simulink model "orthographic_projection_sfchart_tb"  (R2018b)
settings: Solver=FixedStepDiscrete  StartTime=0.0  StopTime=inf  FixedStep=1  RelTol=1e-3
undefined symbols (not defined in the file): lambda0Val, lambdaVec, nIters, numSamples, phi0Val, phiVec, RE
libraries: hdlsllib x10, cordic_rotation_mode x2, simulink x1
settings Model: DataTypeOverride=Off  Creator=jimjoy  LastModifiedBy=tbryan
settings DataIOCC: SaveFormat=StructureWithTime  SaveOutput=off  DSMLogging=off  SaveTime=off  ReturnWorkspaceOutputs=on
settings OptimizationCC: BlockReduction=off  ConditionallyExecuteInputs=off  DefaultParameterBehavior=Inlined
settings DebuggingCC: AlgebraicLoopMsg=error  SingleTaskRateTransMsg=error  UnderSpecifiedDataTypeMsg=error  UnderSpecifiedDimensionMsg=error
settings HardwareCC: ProdBitPerPointer=32  ProdBitPerSizeT=32  ProdBitPerPtrDiffT=32  ProdLargestAtomicFloat=None  ProdIntDivRoundTo=Undefined  ProdEndianess=Unspecified  ProdWordSize=32  ProdHWDeviceType=ASIC/FPGA->ASIC/FPGA  TargetBitPerLong=64  TargetBitPerPointer=64  TargetBitPerSizeT=64  TargetBitPerPtrDiffT=64  TargetLongLongMode=on  TargetIntDivRoundTo=Zero  TargetEndianess=LittleEndian  TargetWordSize=64  TargetHWDeviceType=Custom Processor->MATLAB Host Computer  ProdEqTarget=off

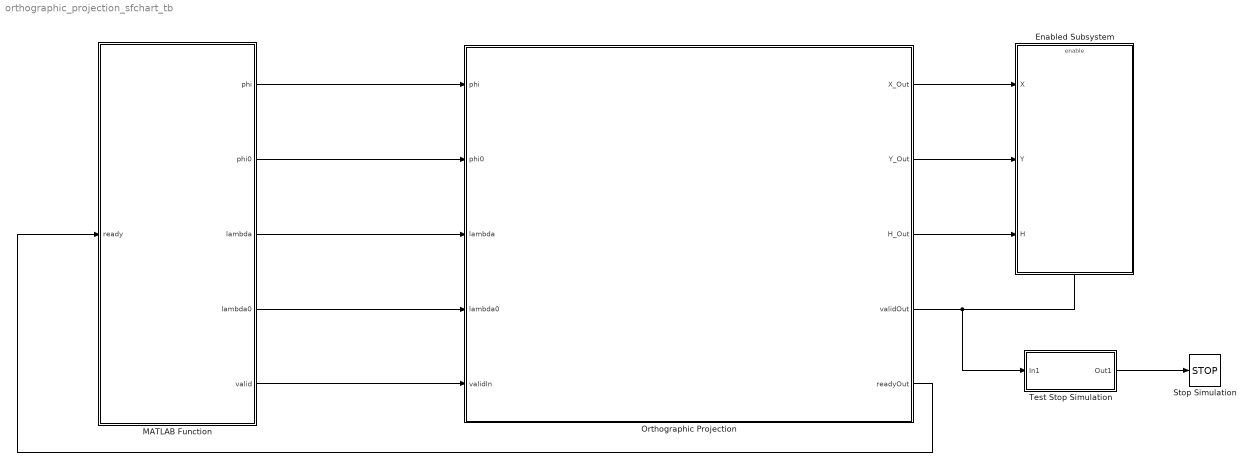
== system orthographic_projection_sfchart_tb ==
  Enabled Subsystem : Subsystem  TreatAsAtomicUnit=on
  MATLAB Function : MATLAB Function  TreatAsAtomicUnit=on  mask{phiVec=phiVec, lambdaVec=lambdaVec, phi0Val=phi0Val, lambda0Val=lambda0Val}
      mask prompts: phiVec "phi"; lambdaVec "lambda"; phi0Val "phi0"; lambda0Val "lambda0"
  Orthographic Projection : Subsystem
  Stop Simulation : Stop
  Test Stop Simulation : Subsystem
  wires:
  Orthographic Projection/1(X_Out) -> Enabled Subsystem/1(X)
  Orthographic Projection/2(Y_Out) -> Enabled Subsystem/2(Y)
  Orthographic Projection/3(H_Out) -> Enabled Subsystem/3(H)
  Orthographic Projection/4(validOut) -> Test Stop Simulation/1(In1), Enabled Subsystem/Enable
  Orthographic Projection/5(readyOut) -> MATLAB Function/1(ready)
  MATLAB Function/5(valid) -> Orthographic Projection/5(validIn)
  MATLAB Function/4(lambda0) -> Orthographic Projection/4(lambda0)
  MATLAB Function/3(lambda) -> Orthographic Projection/3(lambda)
  MATLAB Function/2(phi0) -> Orthographic Projection/2(phi0)
  Test Stop Simulation/1(Out1) -> Stop Simulation/1
  MATLAB Function/1(phi) -> Orthographic Projection/1(phi)

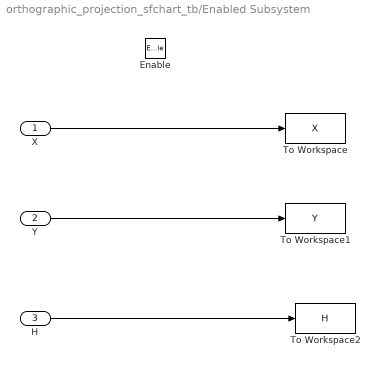
== system orthographic_projection_sfchart_tb/Enabled Subsystem ==
  X : Inport
  Y : Inport  Port=2
  H : Inport  Port=3
  Enable : EnablePort
  To Workspace : ToWorkspace  VariableName=X  SampleTime=-1
      settings: Save2DSignal=2-D array (concatenate along first dimension)
  To Workspace1 : ToWorkspace  VariableName=Y  SampleTime=-1
      settings: Save2DSignal=2-D array (concatenate along first dimension)
  To Workspace2 : ToWorkspace  VariableName=H  SampleTime=-1
      settings: Save2DSignal=2-D array (concatenate along first dimension)
  wires:
  X/1 -> To Workspace/1
  Y/1 -> To Workspace1/1
  H/1 -> To Workspace2/1

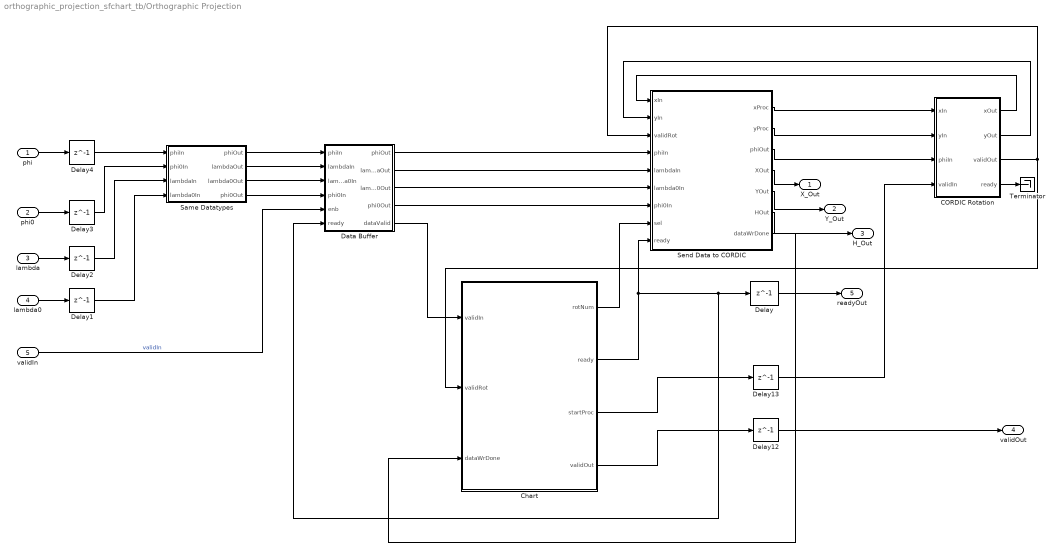
== system orthographic_projection_sfchart_tb/Orthographic Projection ==
  phi : Inport
  phi0 : Inport  Port=2
  lambda : Inport  Port=3
  lambda0 : Inport  Port=4
  validIn : Inport  Port=5
  CORDIC Rotation : Subsystem
  Chart : Stateflow chart  TreatAsAtomicUnit=on
  Data Buffer : Subsystem
  Delay{,1..4,12..13} (7 alike) : Delay  DelayLength=1
  Same Datatypes : Subsystem
  Send Data to CORDIC : Subsystem
  Terminator : Terminator
  X_Out : Outport
  Y_Out : Outport  Port=2
  H_Out : Outport  Port=3
  validOut : Outport  Port=4
  readyOut : Outport  Port=5
  wires:
  CORDIC Rotation/3(validOut) -> Chart/2(validRot), Send Data to CORDIC/3(validRot)
  Chart/4(validOut) -> Delay12/1
  lambda0/1 -> Delay1/1
  phi0/1 -> Delay3/1
  lambda/1 -> Delay2/1
  phi/1 -> Delay4/1
  Delay13/1 -> CORDIC Rotation/4(validIn)
  Send Data to CORDIC/3(phiOut) -> CORDIC Rotation/3(phiIn)
  Send Data to CORDIC/2(yProc) -> CORDIC Rotation/2(yIn)
  Send Data to CORDIC/1(xProc) -> CORDIC Rotation/1(xIn)
  CORDIC Rotation/4(ready) -> Terminator/1
  Delay12/1 -> validOut/1
  Same Datatypes/1(phiOut) -> Data Buffer/1(phiIn)
  Same Datatypes/2(lambdaOut) -> Data Buffer/2(lambdaIn)
  Same Datatypes/3(lambda0Out) -> Data Buffer/3(lambda0In)
  Same Datatypes/4(phi0Out) -> Data Buffer/4(phi0In)
  Delay1/1 -> Same Datatypes/4(lambda0In)
  Delay2/1 -> Same Datatypes/3(lambdaIn)
  Delay3/1 -> Same Datatypes/2(phi0In)
  Delay4/1 -> Same Datatypes/1(phiIn)
  Chart/3(startProc) -> Delay13/1
  CORDIC Rotation/1(xOut) -> Send Data to CORDIC/1(xIn)
  Data Buffer/1(phiOut) -> Send Data to CORDIC/4(phiIn)
  Data Buffer/2(lambdaOut) -> Send Data to CORDIC/5(lambdaIn)
  Data Buffer/3(lambda0Out) -> Send Data to CORDIC/6(lambda0In)
  Data Buffer/4(phi0Out) -> Send Data to CORDIC/7(phi0In)
  CORDIC Rotation/2(yOut) -> Send Data to CORDIC/2(yIn)
  Chart/1(rotNum) -> Send Data to CORDIC/8("sel ")
  Send Data to CORDIC/4(XOut) -> X_Out/1
  Send Data to CORDIC/5(YOut) -> Y_Out/1
  Send Data to CORDIC/6(HOut) -> H_Out/1
  validIn/1 -> Data Buffer/5(enb)  "validIn"
  Data Buffer/5(dataValid) -> Chart/1(validIn)
  Chart/2(ready) -> Data Buffer/6(ready), Delay/1, Send Data to CORDIC/9(ready)
  Delay/1 -> readyOut/1
  Send Data to CORDIC/7(dataWrDone) -> Chart/3(dataWrDone)

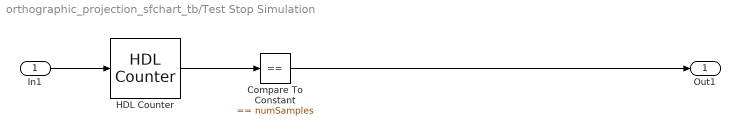
== system orthographic_projection_sfchart_tb/Test Stop Simulation ==
  In1 : Inport
  Compare To Constant : simulink/Logic and Bit Operations/Compare To Constant  relop===  const=numSamples  OutDataTypeStr=boolean
  HDL Counter : hdlsllib/Sources/HDL Counter  CountType=Free running  CountInit=0  CountStep=1  CountMax=25  CountFromType=Initial value  CountFrom=0  CountResetPort=off  CountLoadPort=off  CountEnbPort=on  CountDirPort=off  CountDataType=Unsigned  CountWordLen=nextpow2(numSamples)  CountFracLen=0  CountSampTime=1
      settings: SourceProductName=Simulink
  Out1 : Outport
  wires:
  In1/1 -> HDL Counter/1
  HDL Counter/1 -> Compare To Constant/1
  Compare To Constant/1 -> Out1/1

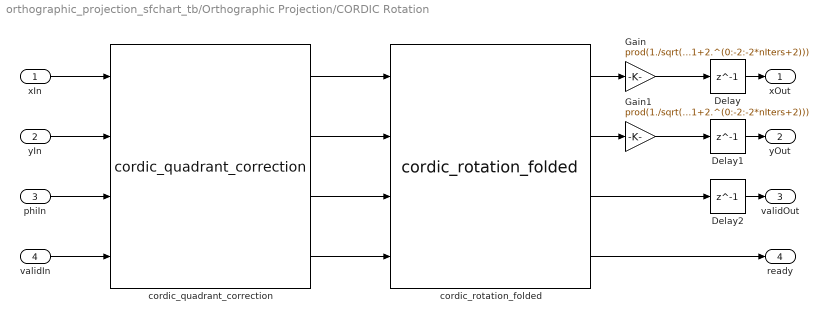
== system orthographic_projection_sfchart_tb/Orthographic Projection/CORDIC Rotation ==
  xIn : Inport
  yIn : Inport  Port=2
  phiIn : Inport  Port=3
  validIn : Inport  Port=4
  Delay : Delay  DelayLength=1
  Delay1 : Delay  DelayLength=1
  Delay2 : Delay  DelayLength=1
  Gain : Gain  Gain=prod(1./sqrt(1+2.^(0:-2:-2*nIters+2)))  OutDataTypeStr=Inherit: Same as input
  Gain1 : Gain  Gain=prod(1./sqrt(1+2.^(0:-2:-2*nIters+2)))  OutDataTypeStr=Inherit: Same as input
  cordic_quadrant_correction : cordic_rotation_mode/cordic_quadrant_correction  SystemSampleTime=-1
  cordic_rotation_folded : cordic_rotation_mode/cordic_rotation_folded  SystemSampleTime=-1
  xOut : Outport
  yOut : Outport  Port=2
  validOut : Outport  Port=3
  ready : Outport  Port=4
  wires:
  Gain1/1 -> Delay1/1
  cordic_quadrant_correction/1 -> cordic_rotation_folded/1
  cordic_rotation_folded/3 -> Delay2/1
  cordic_rotation_folded/2 -> Gain1/1
  cordic_rotation_folded/1 -> Gain/1
  cordic_quadrant_correction/2 -> cordic_rotation_folded/2
  cordic_quadrant_correction/3 -> cordic_rotation_folded/3
  Gain/1 -> Delay/1
  cordic_quadrant_correction/4 -> cordic_rotation_folded/4
  xIn/1 -> cordic_quadrant_correction/1
  Delay/1 -> xOut/1
  Delay2/1 -> validOut/1
  validIn/1 -> cordic_quadrant_correction/4
  Delay1/1 -> yOut/1
  phiIn/1 -> cordic_quadrant_correction/3
  yIn/1 -> cordic_quadrant_correction/2
  cordic_rotation_folded/4 -> ready/1

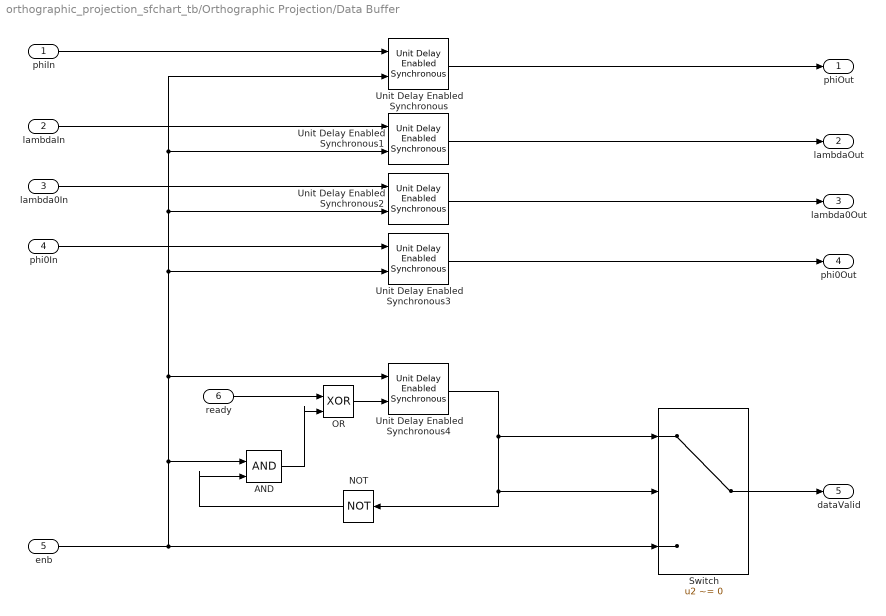
== system orthographic_projection_sfchart_tb/Orthographic Projection/Data Buffer ==
  phiIn : Inport
  lambdaIn : Inport  Port=2
  lambda0In : Inport  Port=3
  phi0In : Inport  Port=4
  enb : Inport  Port=5
  ready : Inport  Port=6
  AND : Logic  IconShape=distinctive  AllPortsSameDT=off  OutDataTypeStr=boolean
  NOT : Logic  Operator=NOT  IconShape=distinctive  AllPortsSameDT=off  OutDataTypeStr=boolean
  OR : Logic  Operator=XOR  IconShape=distinctive  AllPortsSameDT=off  OutDataTypeStr=boolean
  Switch : Switch  Criteria=u2 ~= 0
  Unit Delay Enabled Synchronous{,1..4} (5 alike) : hdlsllib/Discrete/Unit Delay Enabled Synchronous  InitialCondition=0.0  SampleTime=-1
      settings: SourceProductName=Simulink  SourceProductBaseCode=SL
  phiOut : Outport
  lambdaOut : Outport  Port=2
  lambda0Out : Outport  Port=3
  phi0Out : Outport  Port=4
  dataValid : Outport  Port=5
  wires:
  phiIn/1 -> Unit Delay Enabled Synchronous/1
  lambdaIn/1 -> Unit Delay Enabled Synchronous1/1
  lambda0In/1 -> Unit Delay Enabled Synchronous2/1
  phi0In/1 -> Unit Delay Enabled Synchronous3/1
  enb/1 -> AND/1, Unit Delay Enabled Synchronous4/1, Unit Delay Enabled Synchronous3/2, Unit Delay Enabled Synchronous2/2, Unit Delay Enabled Synchronous1/2, Unit Delay Enabled Synchronous/2, Switch/3
  Unit Delay Enabled Synchronous/1 -> phiOut/1
  Unit Delay Enabled Synchronous1/1 -> lambdaOut/1
  Unit Delay Enabled Synchronous2/1 -> lambda0Out/1
  Unit Delay Enabled Synchronous3/1 -> phi0Out/1
  Unit Delay Enabled Synchronous4/1 -> NOT/1, Switch/2, Switch/1
  ready/1 -> OR/1
  OR/1 -> Unit Delay Enabled Synchronous4/2
  AND/1 -> OR/2
  NOT/1 -> AND/2
  Switch/1 -> dataValid/1

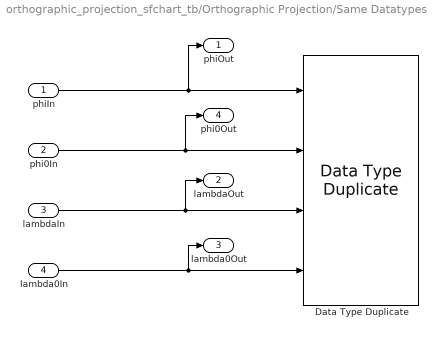
== system orthographic_projection_sfchart_tb/Orthographic Projection/Same Datatypes ==
  phiIn : Inport
  phi0In : Inport  Port=2
  lambdaIn : Inport  Port=3
  lambda0In : Inport  Port=4
  Data Type Duplicate : DataTypeDuplicate  NumInputPorts=4
  phiOut : Outport
  lambdaOut : Outport  Port=2
  lambda0Out : Outport  Port=3
  phi0Out : Outport  Port=4
  wires:
  lambdaIn/1 -> lambdaOut/1, Data Type Duplicate/3
  phiIn/1 -> Data Type Duplicate/1, phiOut/1
  lambda0In/1 -> lambda0Out/1, Data Type Duplicate/4
  phi0In/1 -> phi0Out/1, Data Type Duplicate/2

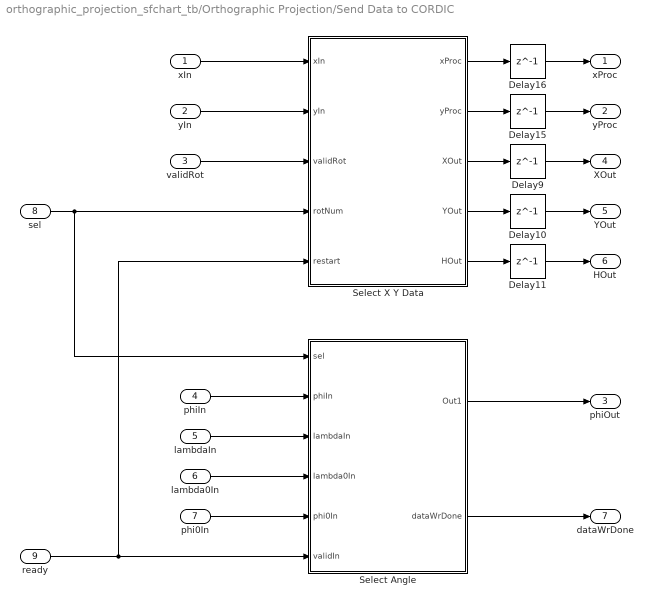
== system orthographic_projection_sfchart_tb/Orthographic Projection/Send Data to CORDIC ==
  xIn : Inport
  yIn : Inport  Port=2
  validRot : Inport  Port=3
  phiIn : Inport  Port=4
  lambdaIn : Inport  Port=5
  lambda0In : Inport  Port=6
  phi0In : Inport  Port=7
  "sel " : Inport  Port=8
  ready : Inport  Port=9
  Delay{9..11,15..16} (5 alike) : Delay  DelayLength=1
  Select Angle : Subsystem
  Select X Y Data : Subsystem  mask{RE=RE}
      mask prompts: RE "Radius of the Earth"
  xProc : Outport
  yProc : Outport  Port=2
  phiOut : Outport  Port=3
  XOut : Outport  Port=4
  YOut : Outport  Port=5
  HOut : Outport  Port=6
  dataWrDone : Outport  Port=7
  wires:
  "sel "/1 -> Select Angle/1(sel), Select X Y Data/4(rotNum)
  ready/1 -> Select X Y Data/5(restart), Select Angle/6("validIn ")
  phiIn/1 -> Select Angle/2(phiIn)
  lambdaIn/1 -> Select Angle/3(lambdaIn)
  lambda0In/1 -> Select Angle/4(lambda0In)
  phi0In/1 -> Select Angle/5(phi0In)
  Select X Y Data/1(xProc) -> Delay16/1
  xIn/1 -> Select X Y Data/1(xIn)
  Select X Y Data/2(yProc) -> Delay15/1
  yIn/1 -> Select X Y Data/2(yIn)
  validRot/1 -> Select X Y Data/3(validRot)
  Select X Y Data/3(XOut) -> Delay9/1
  Select X Y Data/5(HOut) -> Delay11/1
  Select X Y Data/4(YOut) -> Delay10/1
  Delay10/1 -> YOut/1
  Delay9/1 -> XOut/1
  Delay11/1 -> HOut/1
  Delay16/1 -> xProc/1
  Delay15/1 -> yProc/1
  Select Angle/1(Out1) -> phiOut/1
  Select Angle/2(dataWrDone) -> dataWrDone/1

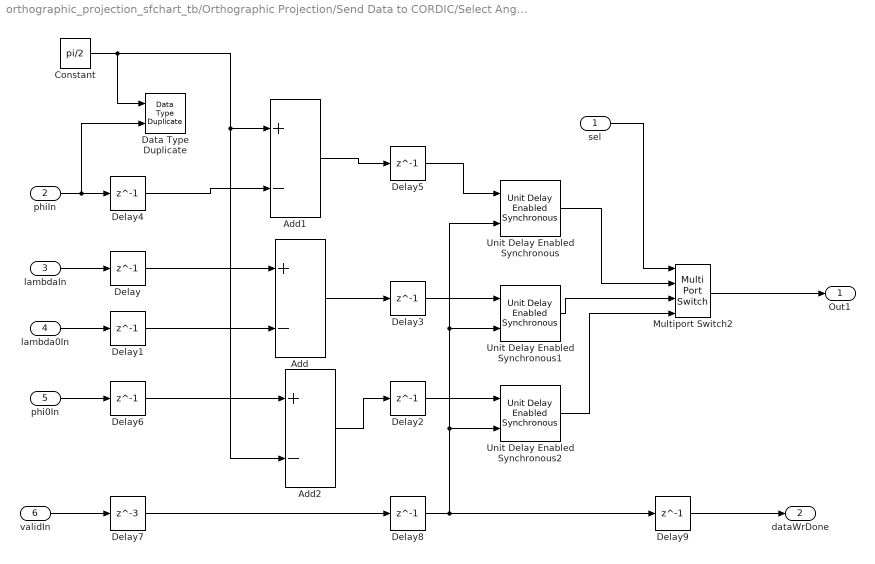
== system orthographic_projection_sfchart_tb/Orthographic Projection/Send Data to CORDIC/Select Angle ==
  sel : Inport
  phiIn : Inport  Port=2
  lambdaIn : Inport  Port=3
  lambda0In : Inport  Port=4
  phi0In : Inport  Port=5
  "validIn " : Inport  Port=6
  Add : Sum  Inputs=+-
  Add1 : Sum  Inputs=+-
  Add2 : Sum  Inputs=+-
  Constant : Constant  Value=pi/2  OutDataTypeStr=Inherit: Inherit via back propagation
  Data Type Duplicate : DataTypeDuplicate
  Delay{,1..6,8..9} (9 alike) : Delay  DelayLength=1
  Delay7 : Delay  DelayLength=3
  Multiport Switch2 : MultiPortSwitch  DataPortOrder=Zero-based contiguous  zeroidx=on
  Unit Delay Enabled Synchronous : hdlsllib/Discrete/Unit Delay Enabled Synchronous  InitialCondition=0.0  SampleTime=-1
      settings: SourceProductName=Simulink  SourceProductBaseCode=SL
  Unit Delay Enabled Synchronous1 : hdlsllib/Discrete/Unit Delay Enabled Synchronous  InitialCondition=0.0  SampleTime=-1
      settings: SourceProductName=Simulink  SourceProductBaseCode=SL
  Unit Delay Enabled Synchronous2 : hdlsllib/Discrete/Unit Delay Enabled Synchronous  InitialCondition=0.0  SampleTime=-1
      settings: SourceProductName=Simulink  SourceProductBaseCode=SL
  Out1 : Outport
  dataWrDone : Outport  Port=2
  wires:
  Unit Delay Enabled Synchronous/1 -> Multiport Switch2/2
  Unit Delay Enabled Synchronous1/1 -> Multiport Switch2/3
  Unit Delay Enabled Synchronous2/1 -> Multiport Switch2/4
  Multiport Switch2/1 -> Out1/1
  sel/1 -> Multiport Switch2/1
  "validIn "/1 -> Delay7/1
  phi0In/1 -> Delay6/1
  phiIn/1 -> Data Type Duplicate/2, Delay4/1
  lambdaIn/1 -> Delay/1
  lambda0In/1 -> Delay1/1
  Delay/1 -> Add/1
  Delay1/1 -> Add/2
  Add/1 -> Delay3/1
  Add2/1 -> Delay2/1
  Delay2/1 -> Unit Delay Enabled Synchronous2/1
  Delay3/1 -> Unit Delay Enabled Synchronous1/1
  Delay5/1 -> Unit Delay Enabled Synchronous/1
  Delay6/1 -> Add2/1
  Delay7/1 -> Delay8/1
  Delay8/1 -> Delay9/1, Unit Delay Enabled Synchronous/2, Unit Delay Enabled Synchronous1/2, Unit Delay Enabled Synchronous2/2
  Delay9/1 -> dataWrDone/1
  Delay4/1 -> Add1/2
  Add1/1 -> Delay5/1
  Constant/1 -> Data Type Duplicate/1, Add2/2, Add1/1

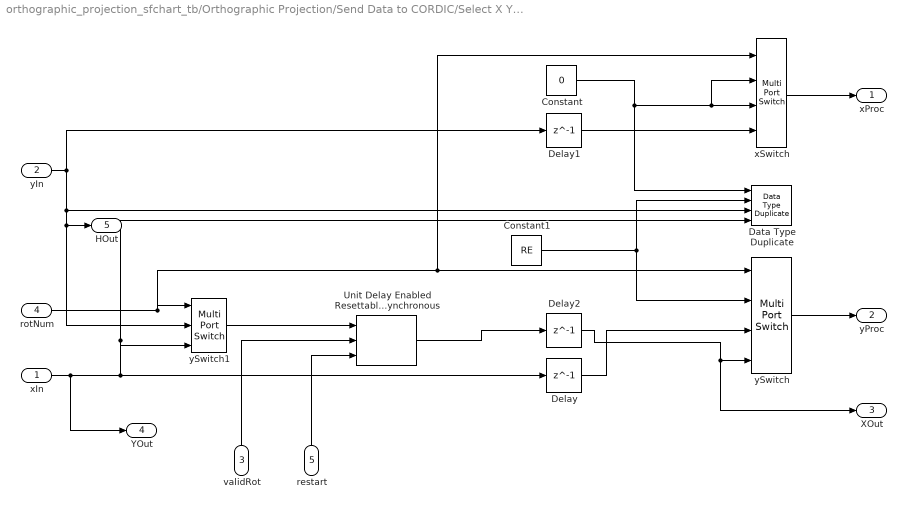
== system orthographic_projection_sfchart_tb/Orthographic Projection/Send Data to CORDIC/Select X Y Data ==
  xIn : Inport
  yIn : Inport  Port=2
  validRot : Inport  Port=3
  rotNum : Inport  Port=4
  restart : Inport  Port=5
  Constant : Constant  Value=0  OutDataTypeStr=Inherit: Inherit via back propagation
  Constant1 : Constant  Value=RE
  Data Type Duplicate : DataTypeDuplicate  NumInputPorts=4
  Delay : Delay  DelayLength=1
  Delay1 : Delay  DelayLength=1
  Delay2 : Delay  DelayLength=1
  Unit Delay Enabled Resettable Synchronous : hdlsllib/Discrete/Unit Delay Enabled Resettable Synchronous  InitialCondition=0.0  SampleTime=-1
      settings: SourceProductName=Simulink  SourceProductBaseCode=SL
  xSwitch : MultiPortSwitch  DataPortOrder=Zero-based contiguous  zeroidx=on
  ySwitch : MultiPortSwitch  DataPortOrder=Zero-based contiguous  zeroidx=on
  ySwitch1 : MultiPortSwitch  DataPortOrder=Zero-based contiguous  Inputs=2  DiagnosticForDefault=None  zeroidx=on
  xProc : Outport
  yProc : Outport  Port=2
  XOut : Outport  Port=3
  YOut : Outport  Port=4
  HOut : Outport  Port=5
  wires:
  ySwitch/1 -> yProc/1
  xSwitch/1 -> xProc/1
  Constant/1 -> Data Type Duplicate/1, xSwitch/3, xSwitch/2
  Constant1/1 -> Data Type Duplicate/2, ySwitch/2
  Unit Delay Enabled Resettable Synchronous/1 -> Delay2/1
  xIn/1 -> Data Type Duplicate/4, ySwitch1/3, Delay/1, YOut/1
  yIn/1 -> Data Type Duplicate/3, ySwitch1/2, HOut/1, Delay1/1
  ySwitch1/1 -> Unit Delay Enabled Resettable Synchronous/1
  rotNum/1 -> ySwitch1/1, ySwitch/1, xSwitch/1
  validRot/1 -> Unit Delay Enabled Resettable Synchronous/2
  restart/1 -> Unit Delay Enabled Resettable Synchronous/3
  Delay/1 -> ySwitch/3
  Delay1/1 -> xSwitch/4
  Delay2/1 -> XOut/1, ySwitch/4

== matlab function orthographic_projection_sfchart_tb/MATLAB Function ==
  data: ready input; phi output; phi0 output; lambda output; lambda0 output; valid output; phiVec parameter; lambdaVec parameter; numSamples parameter; phi0Val parameter; lambda0Val parameter
function [phi, phi0, lambda, lambda0, valid] = getData(ready, phiVec, lambdaVec, numSamples, phi0Val, lambda0Val)
%#codegen

persistent ii 

if isempty(ii)
    ii = 1;
end

phi0 = phi0Val;
lambda0 = lambda0Val;
phi = phiVec(ii);
lambda = lambdaVec(ii);

if ready
   valid = true;
   if ii < numSamples
      ii = ii + 1;
   else
       ii = 1;
   end
else
    valid = false;
end

end

== stateflow chart orthographic_projection_sfchart_tb/Orthographic Projection/Chart ==
  settings: stateMachineType=MEALY_MACHINE  executeAtInitialization=1
  state Controller
    state Init
    state Done
    state Idle
    state Processing
    state ProcessRotResults
    (default) -> Init : {ready = true;}
    Done -> Init : {rotNum = 0; ready = true;validOut = false;}
    Init -> Idle : [validIn]{ready = false;}
    Processing -> Done [order 1] : [validRot && rotNum >= 2]{validOut = true;startProc = false;}
    Idle -> Processing : [dataWrDone]{startProc=true;}
    ProcessRotResults -> Processing : {rotNum++; startProc = true;}
    Processing -> ProcessRotResults [order 2] : [validRot && rotNum < 2]
    Processing -> Processing [order 3] : {startProc = false;}
  data: rotNum output fixdt(0,2,0); ready output boolean; startProc output boolean; validIn input; validRot input; validOut output boolean; dataWrDone input
